simulink model "ukol_5_model_2"  (R2017a)
settings: Solver=VariableStepAuto  StartTime=0.0  StopTime=35  MaxStep=1e-2  RelTol=1e-3
values from neighbouring files (symbols this model uses):
  A = [0 1; -1.44 -0.36]    [ukol_5_script.m]
  B = [0; 1]    [ukol_5_script.m]
  C_1 = [7.2 0]    [ukol_5_script.m]
  D = [0; 0]    [ukol_5_script.m]    (also in ukol_8_script.m = 0; ukol_9_script.m)
  k1 = 0.982    [ukol_5_script.m]    (also in ukol_9_script.m)
  k1_2 = 6.645    [ukol_5_script.m]
  k2 = 1.8188    [ukol_5_script.m]    (also in ukol_9_script.m)
  k2_2 = 3.083    [ukol_5_script.m]
  kI = 3.767    [ukol_5_script.m]
  korekcni_zesileni = 1/0.846    (= 1.18203309693)    [ukol_5_script.m]
settings Model: Creator=tomas  LastModifiedBy=tomas

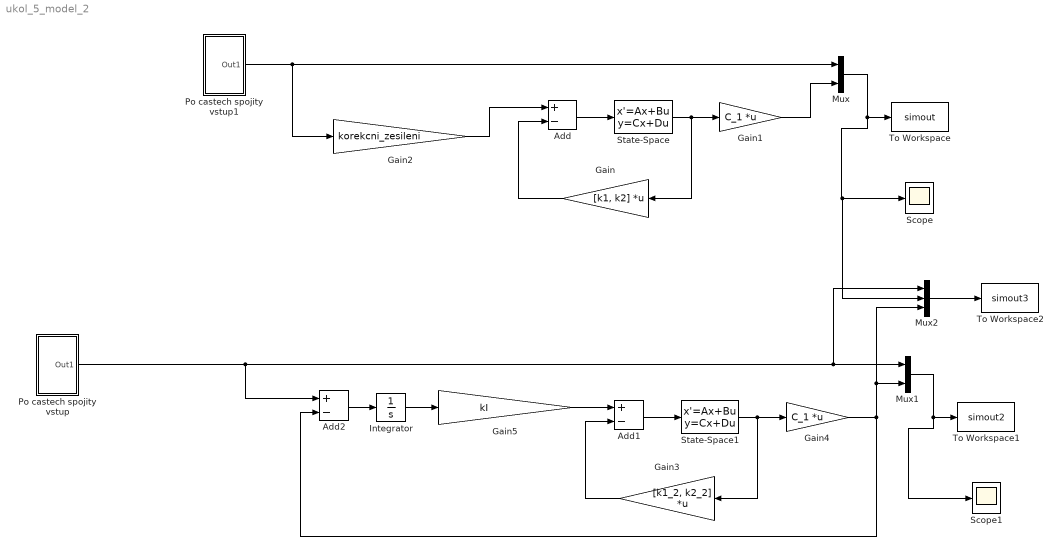
== system ukol_5_model_2 ==
  Add : Sum  Inputs=+-
  Add1 : Sum  Inputs=+-
  Add2 : Sum  Inputs=+-
  Gain : Gain  Gain=[k1, k2]  Multiplication=Matrix(K*u)
  Gain1 : Gain  Gain=C_1  Multiplication=Matrix(K*u)
  Gain2 : Gain  Gain=korekcni_zesileni
  Gain3 : Gain  Gain=[k1_2, k2_2]  Multiplication=Matrix(K*u)
  Gain4 : Gain  Gain=C_1  Multiplication=Matrix(K*u)
  Gain5 : Gain  Gain=kI
  Integrator : Integrator
  Mux : Mux  Inputs=2
  Mux1 : Mux  Inputs=2
  Mux2 : Mux  Inputs=3
  Po castech spojity vstup : Subsystem
  Po castech spojity vstup1 : Subsystem
  Scope : Scope
  Scope1 : Scope
  State-Space : StateSpace  A=A  B=B  C=[1 0; 0 1]  D=D  X0=0
  State-Space1 : StateSpace  A=A  B=B  C=[1 0; 0 1]  D=D  X0=0
  To Workspace : ToWorkspace  VariableName=simout  SaveFormat=Timeseries  SampleTime=-1
  To Workspace1 : ToWorkspace  VariableName=simout2  SaveFormat=Timeseries  SampleTime=-1
  To Workspace2 : ToWorkspace  VariableName=simout3  SaveFormat=Timeseries  SampleTime=-1
  wires:
  State-Space/1 -> Gain/1, Gain1/1
  Add/1 -> State-Space/1
  Gain/1 -> Add/2
  Gain1/1 -> Mux/2
  Mux/1 -> Mux2/2, Scope/1, To Workspace/1
  Gain2/1 -> Add/1
  Gain5/1 -> Add1/1
  Gain4/1 -> Add2/2, Mux2/3, Mux1/2
  State-Space1/1 -> Gain3/1, Gain4/1
  Add1/1 -> State-Space1/1
  Mux1/1 -> Scope1/1, To Workspace1/1
  Gain3/1 -> Add1/2
  Integrator/1 -> Gain5/1
  Add2/1 -> Integrator/1
  Po castech spojity vstup/1(Out1) -> Mux2/1, Mux1/1, Add2/1
  Po castech spojity vstup1/1(Out1) -> Mux/1, Gain2/1
  Mux2/1 -> To Workspace2/1

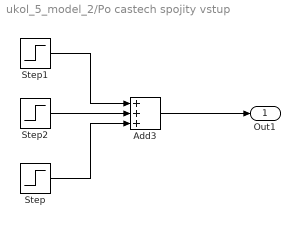
== system ukol_5_model_2/Po castech spojity vstup ==
  Add3 : Sum  Inputs=+++
  Step : Step  SampleTime=0
  Step1 : Step  Time=12  After=-4  SampleTime=0
  Step2 : Step  Time=25  After=8  SampleTime=0
  Out1 : Outport
  wires:
  Step2/1 -> Add3/2
  Step1/1 -> Add3/1
  Step/1 -> Add3/3
  Add3/1 -> Out1/1

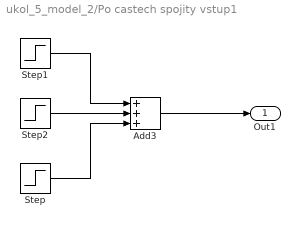
== system ukol_5_model_2/Po castech spojity vstup1 ==
  Add3 : Sum  Inputs=+++
  Step : Step  SampleTime=0
  Step1 : Step  Time=12  After=-4  SampleTime=0
  Step2 : Step  Time=25  After=8  SampleTime=0
  Out1 : Outport
  wires:
  Step2/1 -> Add3/2
  Step/1 -> Add3/3
  Add3/1 -> Out1/1
  Step1/1 -> Add3/1
